simulink model "Steering_Designer"  (R2022a)
settings: Solver=VariableStepAuto  StartTime=0.0  StopTime=1  MaxStep=0.0001  RelTol=1e-3
undefined symbols (not defined in the file): CENTER_STEER_ANGLE_MAX, deadband_angle, S1, S2, S3, S4, steer_slope, theta_left, theta_right, theta_sweep
libraries: dspstat3 x2
settings Model: Creator=Inver  LastModifiedBy=Inver

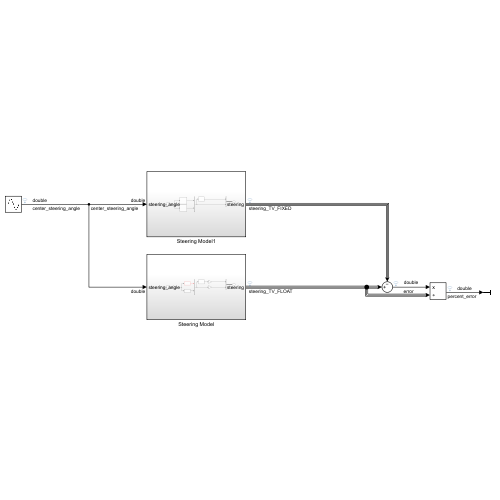
[thumbnail: Simulink's stored preview of the top-level diagram]
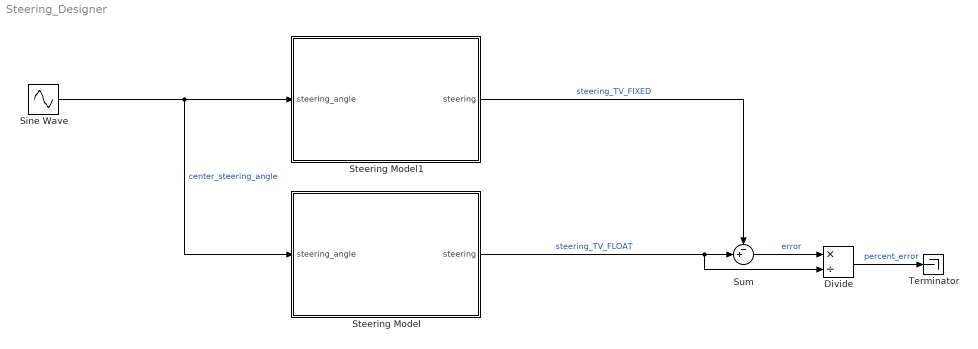
== system Steering_Designer ==
  Divide : Product  Inputs=*/
  Sine Wave : Sin  Amplitude=CENTER_STEER_ANGLE_MAX  Frequency=2*pi  SampleTime=0
  Steering Model : Subsystem
  Steering Model1 : Subsystem
  Sum : Sum  Inputs=-+|
  Terminator : Terminator
  wires:
  Sum/1 -> Divide/1  "error"
  Divide/1 -> Terminator/1  "percent_error"
  Steering Model/1(steering) -> Divide/2, Sum/2  "steering_TV_FLOAT"
  Sine Wave/1 -> Steering Model1/1(steering_angle), Steering Model/1(steering_angle)  "center_steering_angle"
  Steering Model1/1(steering) -> Sum/1  "steering_TV_FIXED"

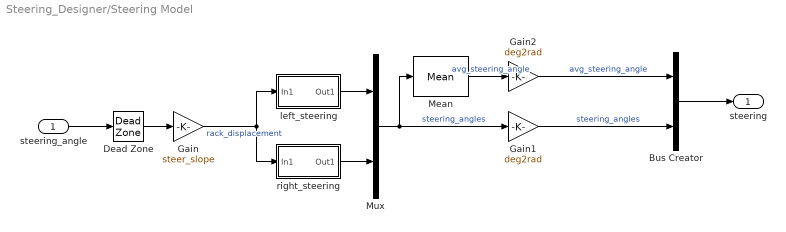
== system Steering_Designer/Steering Model ==
  steering_angle : Inport  OutMin=-130  OutMax=130  OutDataTypeStr=double  LockScale=on
  Bus Creator : BusCreator  Inputs=2
  Dead Zone : DeadZone  LowerValue=-deadband_angle  UpperValue=deadband_angle
  Gain : Gain  Gain=steer_slope  ParamDataTypeStr=double  OutDataTypeStr=double
  Gain1 : Gain  Gain=deg2rad  ParamDataTypeStr=double  OutDataTypeStr=Inherit: Inherit via back propagation
  Gain2 : Gain  Gain=deg2rad  ParamDataTypeStr=double  OutDataTypeStr=Inherit: Inherit via back propagation
  Mean : dspstat3/Mean  run=off  InputProcessing=Columns as channels (frame based)  reset_popup=None  directionMode=Each column  dimension=1  roiEnable=off  roiType=Rectangles  roiPortion=Entire ROI  roiOutput=Individual statistics for each ROI  roiFlag=off  roundingMode=Floor  overflowMode=off  outputDataTypeStr=Inherit: Same as accumulator  outputMin=[]  outputMax=[]  outputLastDataTypeStr=Inherit: Same as accumulator
  Mux : Mux  Inputs=2
  left_steering : Subsystem  Tag=DecoupledSystem
  right_steering : Subsystem  Tag=DecoupledSystem
  steering : Outport  OutDataTypeStr=double  LockScale=on
  wires:
  left_steering/1(Out1) -> Mux/1
  Mean/1 -> Gain2/1  "avg_steering_angle"
  Mux/1 -> Mean/1, Gain1/1  "steering_angles"
  Gain/1 -> left_steering/1(In1), right_steering/1(In1)  "rack_displacement"
  right_steering/1(Out1) -> Mux/2
  Bus Creator/1 -> steering/1
  Gain1/1 -> Bus Creator/2  "steering_angles"
  Gain2/1 -> Bus Creator/1  "avg_steering_angle"
  steering_angle/1 -> Dead Zone/1
  Dead Zone/1 -> Gain/1

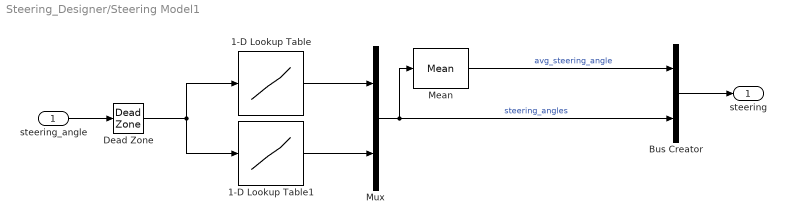
== system Steering_Designer/Steering Model1 ==
  steering_angle : Inport  OutMin=-130  OutMax=130  OutDataTypeStr=double  LockScale=on
  1-D Lookup Table : Lookup_n-D  NumberOfTableDimensions=1  BreakpointsForDimension1=theta_sweep  Table=theta_left  InterpMethod=Cubic spline  InternalRulePriority=Speed  RndMeth=Simplest
  1-D Lookup Table1 : Lookup_n-D  NumberOfTableDimensions=1  BreakpointsForDimension1=theta_sweep  Table=theta_right  InterpMethod=Cubic spline  InternalRulePriority=Speed  RndMeth=Simplest
  Bus Creator : BusCreator  Inputs=2
  Dead Zone : DeadZone  LowerValue=-deadband_angle  UpperValue=deadband_angle
  Mean : dspstat3/Mean  run=off  InputProcessing=Columns as channels (frame based)  reset_popup=None  directionMode=Each column  dimension=1  roiEnable=off  roiType=Rectangles  roiPortion=Entire ROI  roiOutput=Individual statistics for each ROI  roiFlag=off  roundingMode=Floor  overflowMode=off  outputDataTypeStr=Inherit: Same as accumulator  outputMin=[]  outputMax=[]  outputLastDataTypeStr=Inherit: Same as accumulator
  Mux : Mux  Inputs=2
  steering : Outport  OutDataTypeStr=double  LockScale=on
  wires:
  1-D Lookup Table/1 -> Mux/1
  Mean/1 -> Bus Creator/1  "avg_steering_angle"
  Mux/1 -> Bus Creator/2, Mean/1  "steering_angles"
  1-D Lookup Table1/1 -> Mux/2
  Bus Creator/1 -> steering/1
  steering_angle/1 -> Dead Zone/1
  Dead Zone/1 -> 1-D Lookup Table1/1, 1-D Lookup Table/1

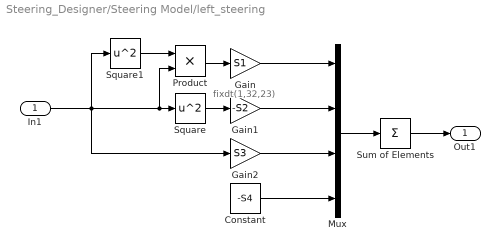
== system Steering_Designer/Steering Model/left_steering ==
  note: fixdt(1,32,23)
  In1 : Inport  OutDataTypeStr=double
  Constant : Constant  Value=-S4  OutDataTypeStr=double
  Gain : Gain  Gain=S1  OutDataTypeStr=double
  Gain1 : Gain  Gain=-S2  OutDataTypeStr=double
  Gain2 : Gain  Gain=S3  OutDataTypeStr=double
  Mux : Mux
  Product : Product  OutDataTypeStr=double
  Square : Math  Operator=square  OutDataTypeStr=double
  Square1 : Math  Operator=square  OutDataTypeStr=double
  Sum of Elements : Sum  Inputs=+  OutDataTypeStr=Inherit: Inherit via back propagation
  Out1 : Outport  OutDataTypeStr=double
  wires:
  Gain2/1 -> Mux/3
  Product/1 -> Gain/1
  Square/1 -> Gain1/1
  Square1/1 -> Product/1
  In1/1 -> Square1/1, Product/2, Square/1, Gain2/1
  Gain1/1 -> Mux/2
  Constant/1 -> Mux/4
  Mux/1 -> Sum of Elements/1
  Gain/1 -> Mux/1
  Sum of Elements/1 -> Out1/1

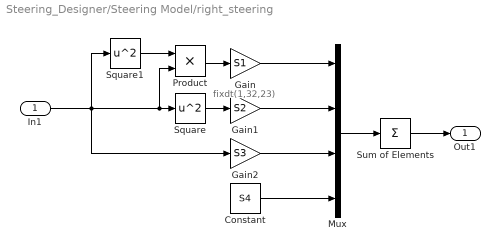
== system Steering_Designer/Steering Model/right_steering ==
  note: fixdt(1,32,23)
  In1 : Inport  OutDataTypeStr=double
  Constant : Constant  Value=S4  OutDataTypeStr=double
  Gain : Gain  Gain=S1  OutDataTypeStr=double
  Gain1 : Gain  Gain=S2  OutDataTypeStr=double
  Gain2 : Gain  Gain=S3  OutDataTypeStr=double
  Mux : Mux
  Product : Product  OutDataTypeStr=double
  Square : Math  Operator=square  OutDataTypeStr=double
  Square1 : Math  Operator=square  OutDataTypeStr=double
  Sum of Elements : Sum  Inputs=+  OutDataTypeStr=Inherit: Inherit via back propagation
  Out1 : Outport  OutDataTypeStr=double
  wires:
  Gain1/1 -> Mux/2
  Gain/1 -> Mux/1
  Gain2/1 -> Mux/3
  Constant/1 -> Mux/4
  Mux/1 -> Sum of Elements/1
  In1/1 -> Square1/1, Product/2, Square/1, Gain2/1
  Square/1 -> Gain1/1
  Product/1 -> Gain/1
  Square1/1 -> Product/1
  Sum of Elements/1 -> Out1/1
